simulink model "BEV_Laengsdynamikmodell_v2"  (R2023b)
settings: configuration reference "SharedConfig" (kept outside this file)
undefined symbols (not defined in the file): acc_cycle_flag, Analyse, battery, battery_builder_rtmsupport, config_battery, config_gearbox, config_Inverter, config_motor, config_vehicle, GB, gcbh, gearbox_map, k_FW, ModuleAssembly1, ModuleType1, motormap, motormap2
libraries: powerlib x37, nesl_utility x18, GD_Batterymodel_NSGAII_1_lib x12, BatteryProtection x9, fl_lib x7, dspstat3 x4, simulink x3, eePmsmCurrentReferenceGen x2, spsControlledCurrentSourceLib x2, spsVoltageMeasurementLib x2, batt_lib x1, BatteryBalancing x1
(part 2 of 6)

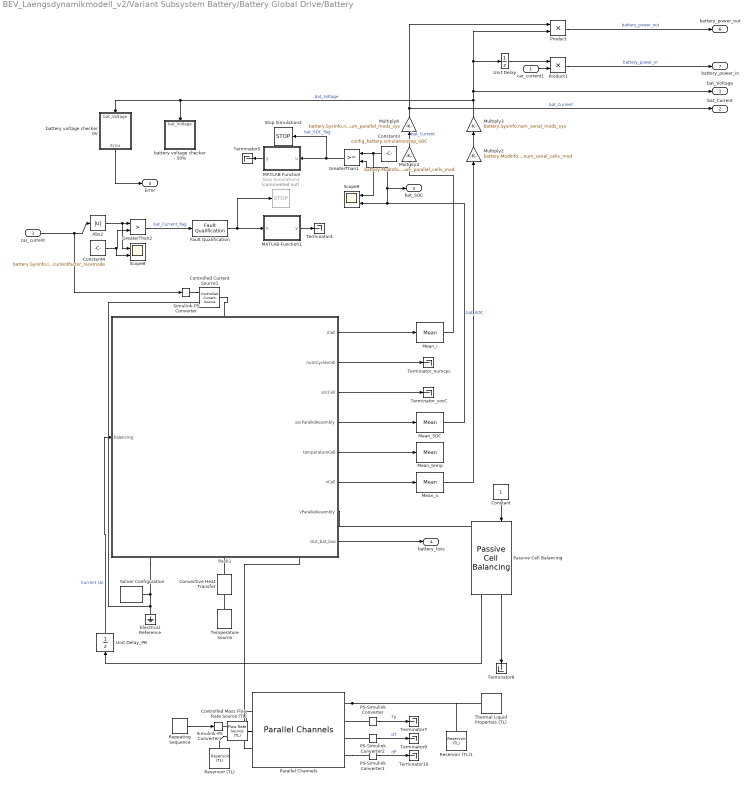
== system BEV_Laengsdynamikmodell_v2/Variant Subsystem Battery/Battery Global Drive/Battery ==
  car_current : Inport
  Abs2 : Abs  SaturateOnIntegerOverflow=off
  Constant : Constant
  Constant3 : Constant  Value=config_battery.simulationstop_SOC
  Constant4 : Constant  Value=battery.SysInfo.I_max_sys * config_battery.overcurrentfactor_racemode
  Controlled Current Source1 : fl_lib/Electrical/Electrical Sources/Controlled Current Source
  Controlled Mass Flow Rate Source (TL) : fl_lib/Thermal Liquid/Sources/Flow Rate Source (TL)  source_type=foundation.enum.constant_controlled.controlled  flow_type=foundation.enum.mass_volumetric_flow.mass  mass_flow=0 kg/s  volumetric_flow=0 m^3/s  power_spec=foundation.enum.power_spec.isentropic  area=0.01 m^2
  Convective Heat Transfer : fl_lib/Thermal/Thermal Elements/Convective Heat Transfer  thermal_type=foundation.enum.constant_variable.constant  area=battery.SysInfo.dim_surface m^2  heat_tr_coeff=20 W/(K*m^2)  min_heat_tr_coeff=1e-3 W/(K*m^2)  T_specify=off  T_priority=None  T=0 K  T_nominal_specify=off  T_nominal_unit=K  T_nominal_value=1  Q_specify=off  Q_priority=None  Q=0 W  Q_nominal_specify=off  Q_nominal_unit=W  Q_nominal_value=1
  Electrical Reference : fl_lib/Electrical/Electrical Elements/Electrical Reference
  Fault Qualification : BatteryProtection/Fault Qualification  QualTime=3  DisqualTime=6  Ts=-1
  GreaterThan1 : RelationalOperator  OutDataTypeStr=boolean  RndMeth=Simplest  InputSameDT=off
  GreaterThan2 : RelationalOperator  Operator=>  OutDataTypeStr=boolean  RndMeth=Simplest  InputSameDT=off
  MATLAB Function : MATLAB Function  TreatAsAtomicUnit=on
  MATLAB Function1 : MATLAB Function  TreatAsAtomicUnit=on
  Mean_SOC : dspstat3/Mean  run=off  InputProcessing=Columns as channels (frame based)  reset_popup=None  directionMode=Entire input  dimension=1  roiEnable=off  roiType=Rectangles  roiPortion=Entire ROI  roiOutput=Individual statistics for each ROI  roiFlag=off  roundingMode=Nearest  overflowMode=off  outputDataTypeStr=Inherit: Same as accumulator  outputMin=[]  outputMax=[]  outputLastDataTypeStr=Inherit: Same as accumulator
  Mean_i : dspstat3/Mean  run=off  InputProcessing=Columns as channels (frame based)  reset_popup=None  directionMode=Entire input  dimension=1  roiEnable=off  roiType=Rectangles  roiPortion=Entire ROI  roiOutput=Individual statistics for each ROI  roiFlag=off  roundingMode=Nearest  overflowMode=off  outputDataTypeStr=Inherit: Same as accumulator  outputMin=[]  outputMax=[]  outputLastDataTypeStr=Inherit: Same as accumulator
  Mean_temp : dspstat3/Mean  run=off  InputProcessing=Columns as channels (frame based)  reset_popup=None  directionMode=Entire input  dimension=1  roiEnable=off  roiType=Rectangles  roiPortion=Entire ROI  roiOutput=Individual statistics for each ROI  roiFlag=off  roundingMode=Nearest  overflowMode=off  outputDataTypeStr=Inherit: Same as accumulator  outputMin=[]  outputMax=[]  outputLastDataTypeStr=Inherit: Same as accumulator
  Mean_v : dspstat3/Mean  run=off  InputProcessing=Columns as channels (frame based)  reset_popup=None  directionMode=Entire input  dimension=1  roiEnable=off  roiType=Rectangles  roiPortion=Entire ROI  roiOutput=Individual statistics for each ROI  roiFlag=off  roundingMode=Nearest  overflowMode=off  outputDataTypeStr=Inherit: Same as accumulator  outputMin=[]  outputMax=[]  outputLastDataTypeStr=Inherit: Same as accumulator
  Multiply2 : Gain  Gain=battery.ModInfo.num_serial_cells_mod
  Multiply3 : Gain  Gain=battery.SysInfo.num_serial_mods_sys
  Multiply4 : Gain  Gain=battery.ModInfo.num_parallel_cells_mod
  Multiply6 : Gain  Gain=battery.SysInfo.num_parallel_mods_sys
  PS-Simulink Converter : nesl_utility/PS-Simulink Converter  PhysicalDomain=network_engine_domain  SubClassName=ps_output  LeftPortType=input  RightPortType=output  PseudoPeriodic=off  Frequencies=[]  VectorFormat=inherit  Unit=inherit  AffineConversion=off
  PS-Simulink Converter1 : nesl_utility/PS-Simulink Converter  PhysicalDomain=network_engine_domain  SubClassName=ps_output  LeftPortType=input  RightPortType=output  PseudoPeriodic=off  Frequencies=[]  VectorFormat=inherit  Unit=inherit  AffineConversion=off
  PS-Simulink Converter2 : nesl_utility/PS-Simulink Converter  PhysicalDomain=network_engine_domain  SubClassName=ps_output  LeftPortType=input  RightPortType=output  PseudoPeriodic=off  Frequencies=[]  VectorFormat=inherit  Unit=inherit  AffineConversion=off
  Pack1 : Subsystem  LoadFcn=battery_builder_rtmsupport('loadfcn',gcbh);
      settings: CopyFcn=battery_builder_rtmsupport('copyfcn',gcbh);  PreCopyFcn=battery_builder_rtmsupport('precopyfcn',gcbh);  PreDeleteFcn=battery_builder_rtmsupport('predeletefcn',gcbh);  PortSchema="{\"entries\":[{\"content\":{\"sides\":[{\"content\":{\"connectorIds\":[\"LConn1\"]},\"type\":\"ConnectorPlacement.EquallySpacedRectSide\",\"uuid\":\"40a787f1-8ebe-41ff-9d70-768a8ef233ef\"},{\"content\":{\"connectorIds\":[\"RConn1\",\"RConn2\",\"RConn3\"],\"side\":\"RIGHT\"},\"type\":\"ConnectorPlacement.EquallySpacedRectSide\",\"uuid\":\"73afe2bc-4ac0-4ad9-926b-4091302672c8\"},{\"content\":{\"connectorIds\":[\"In1\"],\"side\":\"TOP\"},\"type\":\"ConnectorPlacement.EquallySpacedRectSide\",\"uuid\":\"f1f72aa1-a386-4211-9fd1-7dfd903700b9\"},{\"content\":{\"connectorIds\":[\"Out1\",\"Out2\",\"Out3\",\"Out4\",\"Out5\",\"Out6\",\"Out7\",\"Out8\"],\"side\":\"BOTTOM\"},\"type\":\"ConnectorPlacement.EquallySpacedRectSide\",\"uuid\":\"a6cbfe1d-3e62-42c0-b41b-240b72843341\"}]},\"type\":\"ConnectorPlacement.EquallySpacedConnector\",\"uuid\":\"98f8c68d-7fa8-455c-b597-e5213026d8a2\"}],\"packageUris\":[\"http://schema.mathworks.com/mf0/Connector/R2020b\"],\"version\":\"1.0\"}"
      mask Display: image('$imagefile')
  Parallel Channels : batt_lib/Thermal/Parallel Channels  plateConnectivity=simscape.battery.enum.thermal.coolingPlateConnectivity.singleSided  numBattThermalNodes1=1  dimensionThermalNodes1=ones(1, 2)  locationThermalNodes1=ones(1, 2)  numBattThermalNodes2=1  dimensionThermalNodes2=ones(1, 2)  locationThermalNodes2=ones(1, 2)  plateDimX=2  plateDimY=5  plateTh=2e-3 m  plateThCond=20 W/(K*m)  plateDen=2500 kg/m^3  plateCp=447 J/(K*kg)  plateTemp_ini=config_vehicle.ambient_temp K  Re_lam=2000  Re_tur=4000  Nu_lam=3.66  length_add=1e-3 m  shape_factor=64  nChannels=4  selectChannelOrientation=simscape.battery.enum.thermal.coolingChannelsDirection.alongX  channelDia=0.005 m  distributorDia=0.005 m  roughnessPipe=1.5e-05 m
      settings: InternalSimscapePortConfiguration="{\"Bottom\":[],\"Left\":[{\"id\":\"fluid_in\",\"label\":\"fluid_in\",\"type\":\"foundation.thermal_liquid.thermal_liquid\"}],\"Right\":[{\"id\":\"fluid_out\",\"label\":\"fluid_out\",\"type\":\"foundation.thermal_liquid.thermal_liquid\"},{\"id\":\"plotPlateT\",\"label\":\"Tp\",\"type\":\"output\"},{\"id\":\"tempSensor\",\"label\":\"dT\",\"type\":\"output\"},{\"id\":\"presSensor\",\"label\":\"dP\",\"type\":\"output\"}],\"Top\":[{\"id\":\"Side1\",\"label\":\"Surf1\",\"type\":\"foundation.thermal.thermal\"}]}"
  Passive Cell Balancing : BatteryBalancing/Passive Cell Balancing  Threshold=0.2  HysteresisBand=0  Td_on=1  Td_off=1  Ts=-1  dataType=double
  Product : Product
  Product1 : Product
  Repeating Sequence : simulink/Sources/Repeating Sequence  rep_seq_t=[0 2001]  rep_seq_y=[0.1 0.1]
  Reservoir (TL) : fl_lib/Thermal Liquid/Elements/Reservoir (TL)  pressure_spec=foundation.enum.pressure_spec.atmospheric  reservoir_pressure=0.101325 MPa  reservoir_temperature=config_vehicle.ambient_temp K  area=0.01 m^2
  Reservoir (TL)1 : fl_lib/Thermal Liquid/Elements/Reservoir (TL)  pressure_spec=foundation.enum.pressure_spec.atmospheric  reservoir_pressure=0.101325 MPa  reservoir_temperature=config_vehicle.ambient_temp K  area=0.01 m^2
  Scope8 : Scope  NumInputPorts=2
  Scope9 : Scope  NumInputPorts=2
  Simulink-PS Converter : nesl_utility/Simulink-PS Converter  PhysicalDomain=network_engine_domain  SubClassName=ps_input  LeftPortType=input  RightPortType=output  PseudoPeriodic=off  Frequencies=[]  NoiseDistribution=none  NoiseParameters=[]  Unit=1  AffineConversion=off  FilteringAndDerivatives=provide  SimscapeFilterOrder=1  InputFilterTimeConstant=0.001  UdotUserProvided=0
  Simulink-PS Converter1 : nesl_utility/Simulink-PS Converter  PhysicalDomain=network_engine_domain  SubClassName=ps_input  LeftPortType=input  RightPortType=output  PseudoPeriodic=off  Frequencies=[]  NoiseDistribution=none  NoiseParameters=[]  Unit=1  AffineConversion=off  FilteringAndDerivatives=provide  SimscapeFilterOrder=1  InputFilterTimeConstant=0.001  UdotUserProvided=0
  Solver Configuration : nesl_utility/Solver Configuration  PhysicalDomain=network_engine_domain  SubClassName=solver  LeftPortType=input  RightPortType=generic  Tones=[]  Harmonics=[]  SimulateNoise=off  Profile=off  UseLocalSampling=off  EnableSwitchedLinearOptims=on  FrequencyDomain=off  UseCCode=off  RelTol=0.001  AbsTol=0.001  MinStep=1e-09  ToWorkspace=off  RevertToSquareIcSolve=off  NumHomotopyIterations=100  PhasorMode=off  PhasorModeNumHarmonics=1  ConsistencySolver=NEWTON_XTOL_AFTER_FTOL  IndexReductionMethod=DerivativeReplacement  DoDC=off  ResidualTolerance=1e-09  ConsistencyTolSource=GLOBAL  ConsistencyAbsTol=0.001  ConsistencyRelTol=0.001  ConsistencyTolFactor=0.001  UseLocalSolver=on  LocalSolverChoice=NE_BACKWARD_EULER_ADVANCER  ResolveIndetEquations=on  FunctionEvalNumThread=1  LocalSolverSampleTime=1  DoFixedCost=on  MaxNonlinIter=3  MaxModeIter=2  ComputeImpulses=off  ImpulseIterations=2  LinearAlgebra=auto  LinearAlgebraNumThread=0  EquationFormulation=NE_TIME_EF  DelaysMemoryBudget=51200  AutomaticFiltering=on  FilteringTimeConstant=0.001  PartitionStorageMethod=AS_NEEDED  PartitionMemoryBudget=1024  PartitionMethod=ROBUST  MultibodyUseLocalSolver=off  MultibodyLocalSolverChoice=ODE1  MultibodyLocalSolverSampleTime=0.001
  Stop Simulation2 : Stop
  Stop Simulation3 : Stop  Commented=on
  Temperature Source : fl_lib/Thermal/Thermal Sources/Temperature Source  temperature=config_vehicle.ambient_temp K
  Terminator{4..5,7..10} (6 alike) : Terminator
  Terminator_numcyc : Terminator
  Terminator_socC : Terminator
  Thermal Liquid Properties (TL) : SimscapeFluids_lib/Thermal Liquid/Utilities/Thermal Liquid Properties (TL)  fluid_list=fluids.thermal_liquid.utilities.enum.thermal_liquid_fluid_list.water  concentration_param_EG=fluids.thermal_liquid.utilities.enum.thermal_liquid_concentration.volume_fraction  concentration_param_PG=fluids.thermal_liquid.utilities.enum.thermal_liquid_concentration.volume_fraction  c_mass_SW=3.5e-3  c_mass_EG=0.1  c_mass_PG=0.1  c_mass_GL=0.1  c_vol_EG=0.1  c_vol_PG=0.1  beta_const_EG=2.1791 GPa  beta_const_PG=2.1791 GPa  beta_const_GL=2.1791 GPa  p_min_EG=0.01 MPa  p_min_PG=0.01 MPa  p_min_GL=0.01 MPa  p_max_EG=50 MPa  p_max_PG=50 MPa  p_max_GL=50 MPa  p_atm=0.101325 MPa  properties_range_check=simscape.enum.assert.action.error
  Unit Delay : UnitDelay  SampleTime=-1  HasFrameUpgradeWarning=on
  Unit Delay_PB : UnitDelay  SampleTime=-1  HasFrameUpgradeWarning=on
  battery voltage checker - 50% : Subsystem
  battery voltage checker 0V : Subsystem
  car_current1 : InportShadow
  bat_Voltage : Outport
  bat_Current : Outport  Port=2
  bat_SOC : Outport  Port=3
  battery_loss : Outport  Port=4
  Error : Outport  Port=5
  battery_power_out : Outport  Port=6
  battery_power_in : Outport  Port=7
  wires:
  Constant3/1 -> GreaterThan1/1, Scope9/1
  PS-Simulink Converter1/1 -> Terminator10/1  "dP"
  Constant/1 -> Passive Cell Balancing/2
  car_current/1 -> Abs2/1, Simulink-PS Converter/1
  Mean_v/1 -> Multiply2/1
  Multiply3/1 -> bat_Voltage/1, Unit Delay/1, Product/2, battery voltage checker - 50%/1(bat_Voltage), battery voltage checker 0V/1(bat_Voltage)  "bat_Voltage"
  PS-Simulink Converter/1 -> Terminator7/1  "Tp"
  Abs2/1 -> Scope8/1, GreaterThan2/1
  Multiply6/1 -> Product/1, bat_Current/1  "bat_Current"
  Passive Cell Balancing/1 -> Unit Delay_PB/1
  Constant4/1 -> Scope8/2, GreaterThan2/2
  Mean_SOC/1 -> GreaterThan1/2, bat_SOC/1, Scope9/2  "bat_SOC"
  Passive Cell Balancing/2 -> Terminator8/1
  Mean_i/1 -> Multiply4/1
  GreaterThan1/1 -> Stop Simulation2/1, MATLAB Function/1(u)  "bat_SOC_flag"
  GreaterThan2/1 -> Fault Qualification/1  "bat_Current_flag"
  MATLAB Function/1(y) -> Terminator5/1
  MATLAB Function1/1(y) -> Terminator4/1
  Multiply4/1 -> Multiply6/1  "bat_Current"
  battery voltage checker 0V/1(Error) -> Error/1
  Multiply2/1 -> Multiply3/1
  Fault Qualification/1 -> Stop Simulation3/1, MATLAB Function1/1(u)
  Repeating Sequence/1 -> Simulink-PS Converter1/1
  PS-Simulink Converter2/1 -> Terminator9/1  "dT"
  car_current1/1 -> Product1/2
  Unit Delay/1 -> Product1/1
  Product/1 -> battery_power_out/1  "battery_power_out"
  Product1/1 -> battery_power_in/1  "battery_power_in"
  Pack1/1(iCell) -> Mean_i/1
  Pack1/2(numCyclesCell) -> Terminator_numcyc/1
  Pack1/3(socCell) -> Terminator_socC/1
  Pack1/4(socParallelAssembly) -> Mean_SOC/1
  Pack1/5(temperatureCell) -> Mean_temp/1
  Pack1/6(vCell) -> Mean_v/1
  Pack1/7(vParallelAssembly) -> Passive Cell Balancing/1
  Unit Delay_PB/1 -> Pack1/1(balancing)  "Current (A)"
  Pack1/8(Out_bat_loss) -> battery_loss/1
  connections:
  Parallel Channels/RConn1 -- Reservoir (TL)1/LConn1 -- Thermal Liquid Properties (TL)/RConn1
  Temperature Source/LConn1 -- Convective Heat Transfer/RConn1
  Reservoir (TL)/LConn1 -- Controlled Mass Flow Rate Source (TL)/LConn1
  PS-Simulink Converter2/LConn1 -- Parallel Channels/RConn3
  Parallel Channels/RConn4 -- PS-Simulink Converter1/LConn1
  PS-Simulink Converter/LConn1 -- Parallel Channels/RConn2
  Controlled Current Source1/RConn2 -- Electrical Reference/LConn1 -- Solver Configuration/RConn1 -- Pack1/RConn1
  Controlled Mass Flow Rate Source (TL)/RConn1 -- Parallel Channels/LConn1
  Simulink-PS Converter1/RConn1 -- Controlled Mass Flow Rate Source (TL)/LConn2
  Simulink-PS Converter/RConn1 -- Controlled Current Source1/RConn1
  Controlled Current Source1/LConn1 -- Pack1/LConn1
  Pack1/RConn2 -- Convective Heat Transfer/LConn1
  Pack1/RConn3 -- Parallel Channels/LConn2

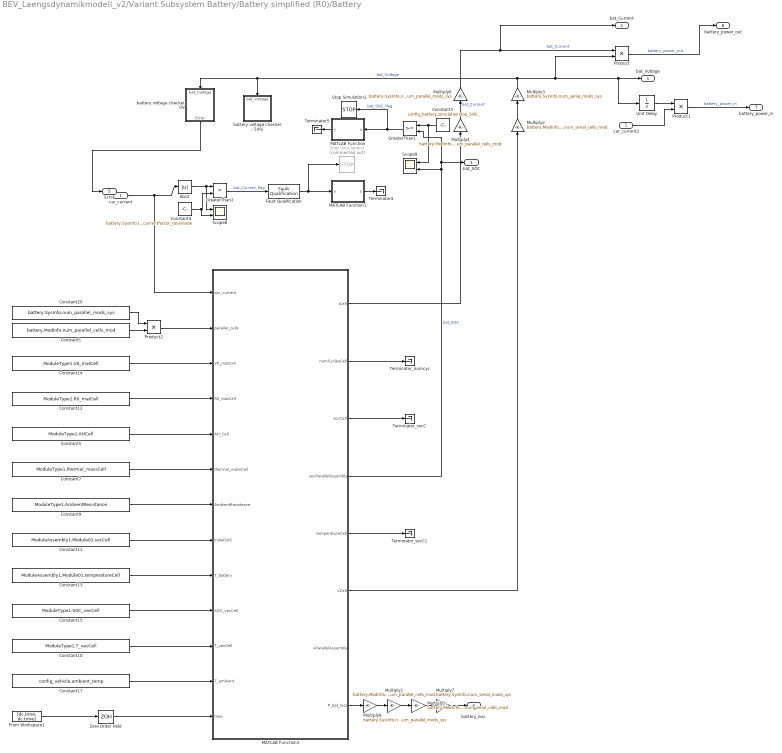
== system BEV_Laengsdynamikmodell_v2/Variant Subsystem Battery/Battery simplified (R0)/Battery ==
  car_current : Inport
  Abs2 : Abs  SaturateOnIntegerOverflow=off
  Constant1 : Constant  Value=battery.ModInfo.num_parallel_cells_mod
  Constant10 : Constant  Value=ModuleType1.T_vecCell
  Constant11 : Constant  Value=ModuleAssembly1.Module01.socCell
  Constant12 : Constant  Value=ModuleType1.R0_matCell
  Constant13 : Constant  Value=ModuleAssembly1.Module01.temperatureCell
  Constant14 : Constant  Value=ModuleType1.V0_matCell
  Constant15 : Constant  Value=ModuleType1.SOC_vecCell
  Constant17 : Constant  Value=config_vehicle.ambient_temp
  Constant20 : Constant  Value=battery.SysInfo.num_parallel_mods_sys
  Constant3 : Constant  Value=config_battery.simulationstop_SOC
  Constant4 : Constant  Value=battery.SysInfo.I_max_sys * config_battery.overcurrentfactor_racemode
  Constant5 : Constant  Value=ModuleType1.AHCell
  Constant7 : Constant  Value=ModuleType1.thermal_massCell
  Constant9 : Constant  Value=ModuleType1.AmbientResistance
  Fault Qualification : BatteryProtection/Fault Qualification  QualTime=3  DisqualTime=6  Ts=-1
  From Workspace1 : FromWorkspace  VariableName=[dc.time, dc.time]
  GreaterThan1 : RelationalOperator  OutDataTypeStr=boolean  RndMeth=Simplest  InputSameDT=off
  GreaterThan2 : RelationalOperator  Operator=>  OutDataTypeStr=boolean  RndMeth=Simplest  InputSameDT=off
  MATLAB Function : MATLAB Function  TreatAsAtomicUnit=on
  MATLAB Function1 : MATLAB Function  TreatAsAtomicUnit=on
  MATLAB Function3 : MATLAB Function  TreatAsAtomicUnit=on
  Multiply1 : Gain  Gain=battery.ModInfo.num_parallel_cells_mod
  Multiply2 : Gain  Gain=battery.ModInfo.num_serial_cells_mod
  Multiply3 : Gain  Gain=battery.SysInfo.num_serial_mods_sys
  Multiply4 : Gain  Gain=battery.ModInfo.num_parallel_cells_mod
  Multiply5 : Gain  Gain=battery.ModInfo.num_serial_cells_mod
  Multiply6 : Gain  Gain=battery.SysInfo.num_parallel_mods_sys
  Multiply7 : Gain  Gain=battery.SysInfo.num_serial_mods_sys
  Multiply8 : Gain  Gain=battery.SysInfo.num_parallel_mods_sys
  Product : Product
  Product1 : Product
  Product2 : Product
  Scope8 : Scope  NumInputPorts=2
  Scope9 : Scope  NumInputPorts=2
  Stop Simulation2 : Stop
  Stop Simulation3 : Stop  Commented=on
  Terminator4 : Terminator
  Terminator5 : Terminator
  Terminator_numcyc : Terminator
  Terminator_socC : Terminator
  Terminator_socC1 : Terminator
  Unit Delay : UnitDelay  SampleTime=-1  HasFrameUpgradeWarning=on
  Zero-Order Hold : ZeroOrderHold  SampleTime=-1
  battery voltage checker - 50% : Subsystem
  battery voltage checker 0V : Subsystem
  car_current2 : InportShadow
  bat_Voltage : Outport
  bat_Current : Outport  Port=2
  bat_SOC : Outport  Port=3
  battery_loss : Outport  Port=4
  Error : Outport  Port=5
  battery_power_out : Outport  Port=6
  battery_power_in : Outport  Port=7
  wires:
  Constant3/1 -> GreaterThan1/1, Scope9/1
  car_current/1 -> MATLAB Function3/1(car_current), Abs2/1
  MATLAB Function3/6(vCell) -> Multiply2/1
  Multiply3/1 -> Product/2, bat_Voltage/1, Unit Delay/1, battery voltage checker - 50%/1(bat_Voltage), battery voltage checker 0V/1(bat_Voltage)  "bat_Voltage"
  Abs2/1 -> Scope8/1, GreaterThan2/1
  Constant4/1 -> Scope8/2, GreaterThan2/2
  MATLAB Function3/4(socParallelAssembly) -> GreaterThan1/2, bat_SOC/1, Scope9/2  "bat_SOC"
  MATLAB Function3/1(iCell) -> Multiply4/1
  GreaterThan1/1 -> Stop Simulation2/1, MATLAB Function/1(u)  "bat_SOC_flag"
  GreaterThan2/1 -> Fault Qualification/1  "bat_Current_flag"
  MATLAB Function/1(y) -> Terminator5/1
  MATLAB Function1/1(y) -> Terminator4/1
  Multiply4/1 -> Multiply6/1  "bat_Current"
  MATLAB Function3/3(socCell) -> Terminator_socC/1
  battery voltage checker 0V/1(Error) -> Error/1
  Multiply2/1 -> Multiply3/1
  Fault Qualification/1 -> Stop Simulation3/1, MATLAB Function1/1(u)
  MATLAB Function3/2(numCyclesCell) -> Terminator_numcyc/1
  MATLAB Function3/5(temperatureCell) -> Terminator_socC1/1
  car_current2/1 -> Product1/2
  Unit Delay/1 -> Product1/1
  Multiply6/1 -> bat_Current/1, Product/1  "bat_Current"
  Product1/1 -> battery_power_in/1  "battery_power_in"
  Product/1 -> battery_power_out/1  "battery_power_out"
  Zero-Order Hold/1 -> MATLAB Function3/13(time)
  From Workspace1/1 -> Zero-Order Hold/1
  Constant5/1 -> MATLAB Function3/5(AH_Cell)
  Constant13/1 -> MATLAB Function3/9(T_battery)
  Constant11/1 -> MATLAB Function3/8(InitialSOC)
  Constant14/1 -> MATLAB Function3/3(V0_matCell)
  Constant12/1 -> MATLAB Function3/4(R0_matCell)
  Constant15/1 -> MATLAB Function3/10(SOC_vecCell)
  Constant7/1 -> MATLAB Function3/6(thermal_massCell)
  Constant10/1 -> MATLAB Function3/11(T_vecCell)
  Constant9/1 -> MATLAB Function3/7(AmbientResistance)
  Constant17/1 -> MATLAB Function3/12(T_ambient)
  Multiply7/1 -> battery_loss/1
  MATLAB Function3/8(P_bat_loss) -> Multiply8/1
  Multiply5/1 -> Multiply7/1
  Multiply1/1 -> Multiply5/1
  Constant1/1 -> Product2/2
  Constant20/1 -> Product2/1
  Product2/1 -> MATLAB Function3/2(parallel_cells)
  Multiply8/1 -> Multiply1/1

== system BEV_Laengsdynamikmodell_v2/Variant Subsystem Gearbox/Gearbox Analytic/Oil Temp ==
  P_V : Inport
  IC : InitialCondition  Value=25
  MATLAB Function : MATLAB Function  TreatAsAtomicUnit=on
  Memory1 : Memory  InitialCondition=config_vehicle.ambient_temp - 273
  Memory2 : Memory  InitialCondition=config_vehicle.ambient_temp - 273
  Scope : Scope
  temp : Outport
  wires:
  MATLAB Function/1(T) -> IC/1  "GB_temp"
  Memory1/1 -> MATLAB Function/1(t)
  P_V/1 -> Memory2/1
  IC/1 -> Scope/1, Memory1/1, temp/1
  Memory2/1 -> MATLAB Function/2(P_V)

== system BEV_Laengsdynamikmodell_v2/Variant Subsystem Gearbox/Gearbox Analytic/Oil Temp Gao ==
  note: entspricht 2pi/60 * 1e-3
  T_wheel : Inport
  rpm_wheel : Inport  Port=2
  MATLAB Function : MATLAB Function  TreatAsAtomicUnit=on
  Memory1 : Memory  InitialCondition=config_vehicle.ambient_temp - 273
  Multiply5 : Gain  Gain=1/9550
  Product2 : Product
  Scope : Scope
  temp : Outport
  wires:
  Product2/1 -> Multiply5/1
  rpm_wheel/1 -> MATLAB Function/3(rpm), Product2/2
  T_wheel/1 -> Product2/1
  MATLAB Function/1(T) -> Scope/1, Memory1/1, temp/1
  Memory1/1 -> MATLAB Function/1(t)
  Multiply5/1 -> MATLAB Function/2(P)

== system BEV_Laengsdynamikmodell_v2/Variant Subsystem Gearbox/Gearbox Analytic/Variant Subsystem Analytic GB ==
  note: 1) Add Subsystem or Model blocks as valid variant choices.
      | 2) You cannot connect blocks at this level. At simulation, connectivity is automatically
      | determined, based on the active variant and port name matching.
  wheel_torque : Inport
  wheel_rpm : Inport  Port=2
  Temp : Inport  Port=3
  Einstufig_Achsparallel : Subsystem  VariantControl=GB_Stufen == 1
  Zweistufig_Achsparallel : Subsystem  VariantControl="GB_Stufen == 2 && GB_Topology == \"achsparallel\""
  Zweistufig_Koaxial : Subsystem  VariantControl="GB_Stufen == 2 && GB_Topology == \"koaxial\""
  P_V : Outport

== system BEV_Laengsdynamikmodell_v2/Variant Subsystem Gearbox/Gearbox Lookup-Table/Oil Temp ==
  P_V : Inport
  IC : InitialCondition  Value=25
  MATLAB Function : MATLAB Function  TreatAsAtomicUnit=on
  Memory1 : Memory  InitialCondition=config_vehicle.ambient_temp - 273
  Memory2 : Memory  InitialCondition=config_vehicle.ambient_temp - 273
  Scope : Scope
  temp : Outport
  wires:
  MATLAB Function/1(T) -> IC/1  "GB_temp"
  Memory1/1 -> MATLAB Function/1(t)
  P_V/1 -> Memory2/1
  IC/1 -> Scope/1, Memory1/1, temp/1
  Memory2/1 -> MATLAB Function/2(P_V)

== system BEV_Laengsdynamikmodell_v2/Variant Subsystem Gearbox/Gearbox Lookup-Table/Oil Temp Gao ==
  note: entspricht 2pi/60 * 1e-3
  T_wheel : Inport
  rpm_wheel : Inport  Port=2
  MATLAB Function : MATLAB Function  TreatAsAtomicUnit=on
  Memory1 : Memory  InitialCondition=config_vehicle.ambient_temp - 273
  Multiply5 : Gain  Gain=1/9550
  Product2 : Product
  Scope : Scope
  temp : Outport
  wires:
  Product2/1 -> Multiply5/1
  rpm_wheel/1 -> MATLAB Function/3(rpm), Product2/2
  T_wheel/1 -> Product2/1
  MATLAB Function/1(T) -> Scope/1, Memory1/1, temp/1
  Memory1/1 -> MATLAB Function/1(t)
  Multiply5/1 -> MATLAB Function/2(P)

== system BEV_Laengsdynamikmodell_v2/Variant Subsystem Gearbox/Gearbox Lookup-Table/Variant Subsystem ==
  note: 1) Add Subsystem or Model blocks as valid variant choices.
      | 2) You cannot connect blocks at this level. At simulation, connectivity is automatically
      | determined, based on the active variant and port name matching.
  wheel_torque : Inport
  wheel_rpm : Inport  Port=2
  Temp : Inport  Port=3
  ETA_map : Subsystem  VariantControl="gearbox_map.map_type == \"Eta\""
  LOSS_map : Subsystem  VariantControl="gearbox_map.map_type == \"Loss\""
  loss_lockup : Outport
  gearbox_efficiency : Outport  Port=2
  gearbox_rpm : Outport  Port=3
  gearbox_torque : Outport  Port=4

== system BEV_Laengsdynamikmodell_v2/Variant Subsystem Inverter/Inverter Analytic/Variant Subsystem ==
  note: 1) Add Subsystem or Model blocks as valid variant choices.
      | 2) You cannot connect blocks at this level. At simulation, connectivity is automatically
      | determined, based on the active variant and port name matching.
  udc : Inport
  rpm : Inport  Port=2
  torque : Inport  Port=3
  terminal_power : Inport  Port=4
  IM_Inverter_IGBT_Analytic : Subsystem  VariantControl=Mode_IM_IGBT
  IM_Inverter_SiC-MOSFET_Analytic : Subsystem  VariantControl=Mode_IM_MOSFET
  PMSM_Inverter_IBGT_Analytic : Subsystem  VariantControl=Mode_PSM_IGBT
  PMSM_Inverter_SiC-MOSFET_Analytic : Subsystem  VariantControl=Mode_PSM_MOSFET
  Conduction_and_Switching_loss : Outport
  idc : Outport  Port=2
  P_inv_total : Outport  Port=3
  P_mot_elec : Outport  Port=4

== system BEV_Laengsdynamikmodell_v2/Variant Subsystem Motor/Motor Analytic/Friction & Windage ==
  note: Gleichung für mechanische Verlustleistung:
      | P_FW = k_FW * n^2.5
  gearbox_rpm : Inport
  Constant : Constant  Value=2.5
  Constant1 : Constant  Value=0
  Constant5 : Constant  Value=k_FW
  Gain : Gain  Gain=2*pi/60
  In2 : InportShadow
  Power : Math  Operator=pow
  Product : Product
  Product2 : Product  Inputs=*/
  Switch : Switch  Criteria=u2 > Threshold  SaturateOnIntegerOverflow=off  InputSameDT=off
  friction torque : Outport
  wires:
  gearbox_rpm/1 -> Power/1  "n_gearbox"
  Constant/1 -> Power/2  "exponent"
  Power/1 -> Product/1
  Constant5/1 -> Product/2
  Product/1 -> Product2/1  "mech powerloss"
  Product2/1 -> Switch/1  "torque"
  In2/1 -> Gain/1  "n_gearbox"
  Gain/1 -> Product2/2, Switch/2
  Switch/1 -> friction torque/1
  Constant1/1 -> Switch/3

== system BEV_Laengsdynamikmodell_v2/Variant Subsystem Motor/Motor Const/Friction & Windage ==
  note: Gleichung für mechanische Verlustleistung:
      | P_FW = k_FW * n^2.5
  gearbox_rpm : Inport
  Constant : Constant  Value=2.5
  Constant1 : Constant  Value=0
  Constant5 : Constant  Value=k_FW
  Gain : Gain  Gain=2*pi/60
  In2 : InportShadow
  Power : Math  Operator=pow
  Product : Product
  Product2 : Product  Inputs=*/
  Switch : Switch  Criteria=u2 > Threshold  SaturateOnIntegerOverflow=off  InputSameDT=off
  friction torque : Outport
  wires:
  gearbox_rpm/1 -> Power/1  "n_gearbox"
  Constant/1 -> Power/2  "exponent"
  Power/1 -> Product/1
  Constant5/1 -> Product/2
  Product/1 -> Product2/1  "mech powerloss"
  Product2/1 -> Switch/1  "torque"
  In2/1 -> Gain/1  "n_gearbox"
  Gain/1 -> Product2/2, Switch/2
  Switch/1 -> friction torque/1
  Constant1/1 -> Switch/3

== system BEV_Laengsdynamikmodell_v2/Variant Subsystem Motor/Motor Lookup-Table/Friction & Windage ==
  note: Gleichung für mechanische Verlustleistung:
      | P_FW = k_FW * n^2.5
  gearbox_rpm : Inport
  Constant : Constant  Value=2.5
  Constant1 : Constant  Value=0
  Constant5 : Constant  Value=k_FW
  Gain : Gain  Gain=2*pi/60
  In2 : InportShadow
  Power : Math  Operator=pow
  Product : Product
  Product2 : Product  Inputs=*/
  Switch : Switch  Criteria=u2 > Threshold  SaturateOnIntegerOverflow=off  InputSameDT=off
  friction torque : Outport
  wires:
  gearbox_rpm/1 -> Power/1  "n_gearbox"
  Constant/1 -> Power/2  "exponent"
  Power/1 -> Product/1
  Constant5/1 -> Product/2
  Product/1 -> Product2/1  "mech powerloss"
  Product2/1 -> Switch/1  "torque"
  In2/1 -> Gain/1  "n_gearbox"
  Gain/1 -> Product2/2, Switch/2
  Switch/1 -> friction torque/1
  Constant1/1 -> Switch/3

== system BEV_Laengsdynamikmodell_v2/Variant Subsystem Motor/Motor Lookup-TableOneMotor/Friction & Windage ==
  note: Gleichung für mechanische Verlustleistung:
      | P_FW = k_FW * n^2.5
  gearbox_rpm : Inport
  Constant : Constant  Value=2.5
  Constant1 : Constant  Value=0
  Constant5 : Constant  Value=k_FW
  Gain : Gain  Gain=2*pi/60
  In2 : InportShadow
  Power : Math  Operator=pow
  Product : Product
  Product2 : Product  Inputs=*/
  Switch : Switch  Criteria=u2 > Threshold  SaturateOnIntegerOverflow=off  InputSameDT=off
  friction torque : Outport
  wires:
  gearbox_rpm/1 -> Power/1  "n_gearbox"
  Constant/1 -> Power/2  "exponent"
  Power/1 -> Product/1
  Constant5/1 -> Product/2
  Product/1 -> Product2/1  "mech powerloss"
  Product2/1 -> Switch/1  "torque"
  In2/1 -> Gain/1  "n_gearbox"
  Gain/1 -> Product2/2, Switch/2
  Switch/1 -> friction torque/1
  Constant1/1 -> Switch/3

== system BEV_Laengsdynamikmodell_v2/Variant Subsystem Battery/Battery Analytic (RC3)/Battery/battery voltage checker - 50% ==
  bat_Voltage : Inport
  Constant : Constant  Value=acc_cycle_flag
  Constant5 : Constant  Value=0.5 * battery.SysInfo.U_max_sys
  Data Type Conversion : DataTypeConversion  OutDataTypeStr=double  SaturateOnIntegerOverflow=off  RndMeth=Floor
  Fault Qualification : BatteryProtection/Fault Qualification  QualTime=2  DisqualTime=4  Ts=-1
  GreaterThan3 : RelationalOperator  Operator=>  OutDataTypeStr=boolean  RndMeth=Simplest  InputSameDT=off
  MATLAB Function2 : MATLAB Function  TreatAsAtomicUnit=on
  Stop Simulation : Stop
  Unit Delay : UnitDelay  SampleTime=-1  HasFrameUpgradeWarning=on
  wires:
  Constant/1 -> MATLAB Function2/3(z)
  Fault Qualification/1 -> MATLAB Function2/1(u)
  MATLAB Function2/2(st) -> Stop Simulation/1
  Data Type Conversion/1 -> MATLAB Function2/2(d)
  Unit Delay/1 -> Data Type Conversion/1
  MATLAB Function2/1(y) -> Unit Delay/1
  bat_Voltage/1 -> GreaterThan3/2
  GreaterThan3/1 -> Fault Qualification/1
  Constant5/1 -> GreaterThan3/1

== system BEV_Laengsdynamikmodell_v2/Variant Subsystem Battery/Battery Analytic (RC3)/Battery/battery voltage checker 0V ==
  bat_Voltage : Inport
  Constant7 : Constant  Value=0
  Fault Qualification1 : BatteryProtection/Fault Qualification  QualTime=1  DisqualTime=3  Ts=-1
  GreaterThan4 : RelationalOperator  Operator=>  OutDataTypeStr=boolean  RndMeth=Simplest  InputSameDT=off
  Error : Outport
  wires:
  Fault Qualification1/1 -> Error/1
  bat_Voltage/1 -> GreaterThan4/2
  GreaterThan4/1 -> Fault Qualification1/1
  Constant7/1 -> GreaterThan4/1

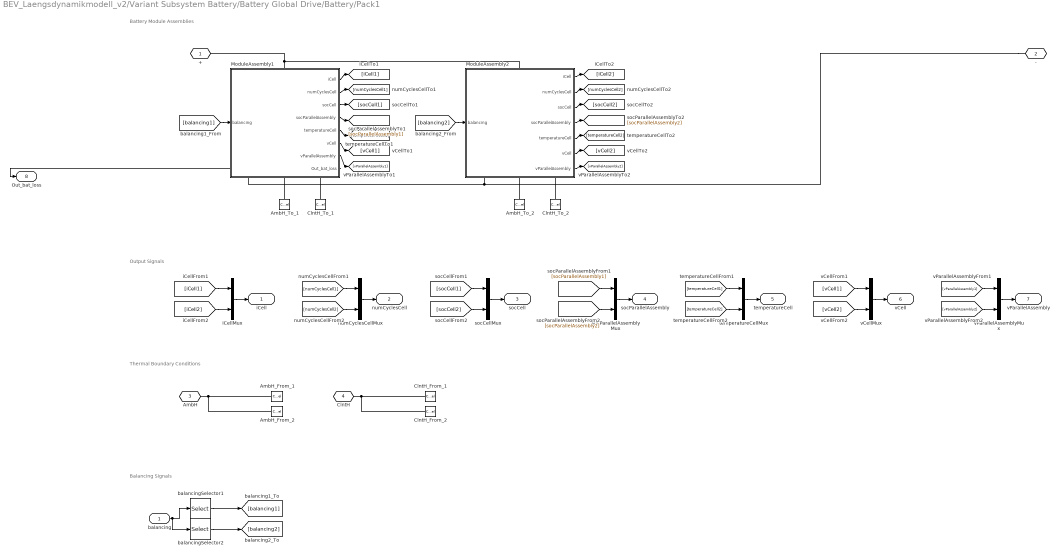
== system BEV_Laengsdynamikmodell_v2/Variant Subsystem Battery/Battery Global Drive/Battery/Pack1 ==
  note: Balancing Signals
  note: Thermal Boundary Conditions
  note: Output Signals
  note: Battery Module Assemblies
  balancing : Inport  PortDimensions=216
  AmbH_From_1 : ConnectionLabel  Label=ambH_1
  AmbH_From_2 : ConnectionLabel  Label=ambH_2
  AmbH_To_1 : ConnectionLabel  Label=ambH_1
  AmbH_To_2 : ConnectionLabel  Label=ambH_2
  ClntH_From_1 : ConnectionLabel  Label=clntH_1
  ClntH_From_2 : ConnectionLabel  Label=clntH_2
  ClntH_To_1 : ConnectionLabel  Label=clntH_1
  ClntH_To_2 : ConnectionLabel  Label=clntH_2
  ModuleAssembly1 : Subsystem  LoadFcn=battery_builder_rtmsupport('loadfcn',gcbh);
      settings: CopyFcn=battery_builder_rtmsupport('copyfcn',gcbh);  PreCopyFcn=battery_builder_rtmsupport('precopyfcn',gcbh);  PreDeleteFcn=battery_builder_rtmsupport('predeletefcn',gcbh);  PortSchema="{\"entries\":[{\"content\":{\"sides\":[{\"content\":{\"connectorIds\":[\"LConn1\"]},\"type\":\"ConnectorPlacement.EquallySpacedRectSide\",\"uuid\":\"40a787f1-8ebe-41ff-9d70-768a8ef233ef\"},{\"content\":{\"connectorIds\":[\"RConn1\",\"RConn2\",\"RConn3\"],\"side\":\"RIGHT\"},\"type\":\"ConnectorPlacement.EquallySpacedRectSide\",\"uuid\":\"73afe2bc-4ac0-4ad9-926b-4091302672c8\"},{\"content\":{\"connectorIds\":[\"In1\"],\"side\":\"TOP\"},\"type\":\"ConnectorPlacement.EquallySpacedRectSide\",\"uuid\":\"f1f72aa1-a386-4211-9fd1-7dfd903700b9\"},{\"content\":{\"connectorIds\":[\"Out1\",\"Out2\",\"Out3\",\"Out4\",\"Out5\",\"Out6\",\"Out7\",\"Out8\"],\"side\":\"BOTTOM\"},\"type\":\"ConnectorPlacement.EquallySpacedRectSide\",\"uuid\":\"00ff99ce-51a0-4b29-8d0f-02bd4eb71b30\"}]},\"type\":\"ConnectorPlacement.EquallySpacedConnector\",\"uuid\":\"98f8c68d-7fa8-455c-b597-e5213026d8a2\"}],\"packageUris\":[\"http://schema.mathworks.com/mf0/Connector/R2020b\"],\"version\":\"1.0\"}"
      mask Display: image('$imagefile')
  ModuleAssembly2 : Subsystem  LoadFcn=battery_builder_rtmsupport('loadfcn',gcbh);
      settings: CopyFcn=battery_builder_rtmsupport('copyfcn',gcbh);  PreCopyFcn=battery_builder_rtmsupport('precopyfcn',gcbh);  PreDeleteFcn=battery_builder_rtmsupport('predeletefcn',gcbh);  PortSchema="{\"entries\":[{\"content\":{\"sides\":[{\"content\":{\"connectorIds\":[\"LConn1\"]},\"type\":\"ConnectorPlacement.EquallySpacedRectSide\",\"uuid\":\"40a787f1-8ebe-41ff-9d70-768a8ef233ef\"},{\"content\":{\"connectorIds\":[\"RConn1\",\"RConn2\",\"RConn3\"],\"side\":\"RIGHT\"},\"type\":\"ConnectorPlacement.EquallySpacedRectSide\",\"uuid\":\"73afe2bc-4ac0-4ad9-926b-4091302672c8\"},{\"content\":{\"connectorIds\":[\"In1\"],\"side\":\"TOP\"},\"type\":\"ConnectorPlacement.EquallySpacedRectSide\",\"uuid\":\"f1f72aa1-a386-4211-9fd1-7dfd903700b9\"},{\"content\":{\"connectorIds\":[\"Out1\",\"Out2\",\"Out3\",\"Out4\",\"Out5\",\"Out6\",\"Out7\"],\"side\":\"BOTTOM\"},\"type\":\"ConnectorPlacement.EquallySpacedRectSide\",\"uuid\":\"00ff99ce-51a0-4b29-8d0f-02bd4eb71b30\"}]},\"type\":\"ConnectorPlacement.EquallySpacedConnector\",\"uuid\":\"98f8c68d-7fa8-455c-b597-e5213026d8a2\"}],\"packageUris\":[\"http://schema.mathworks.com/mf0/Connector/R2020b\"],\"version\":\"1.0\"}"
      mask Display: image('$imagefile')
  balancingSelector1 : Selector  InputPortWidth=216  IndexOptions=Index vector (dialog)  Indices="[1    2    3    4    5    6    7    8    9   10   11   12   13   14   15   16   17   18   19   20   21   22   23   24   25   26   27   28   29   30   31   32   33   34   35   36   37   38   39   40   41   42   43   44   45   46   47   48   49   50   51   52   53   54   55   56   57   58   59   60   61   62   63   64   65   66   67   68   69   70   71   72   73   74   75   76   77   78   79   80   81   82   83   84   85   86   87   88   89   90   91   92   93   94   95   96   97   98   99  100  101  102  103  104  105  106  107  108]"  OutputSizes=1
  balancingSelector2 : Selector  InputPortWidth=216  IndexOptions=Index vector (dialog)  Indices="[109  110  111  112  113  114  115  116  117  118  119  120  121  122  123  124  125  126  127  128  129  130  131  132  133  134  135  136  137  138  139  140  141  142  143  144  145  146  147  148  149  150  151  152  153  154  155  156  157  158  159  160  161  162  163  164  165  166  167  168  169  170  171  172  173  174  175  176  177  178  179  180  181  182  183  184  185  186  187  188  189  190  191  192  193  194  195  196  197  198  199  200  201  202  203  204  205  206  207  208  209  210  211  212  213  214  215  216]"  OutputSizes=1
  iCellMux : Mux  Inputs=2
  numCyclesCellMux : Mux  Inputs=2
  socCellMux : Mux  Inputs=2
  socParallelAssemblyMux : Mux  Inputs=2
  temperatureCellMux : Mux  Inputs=2
  vCellMux : Mux  Inputs=2
  vParallelAssemblyMux : Mux  Inputs=2
  + : PMIOPort  Side=Left
  - : PMIOPort  Port=2  Side=Right
  AmbH : PMIOPort  Port=3  Side=Right  ConnectionType=Connection: foundation.thermal.thermal
  ClntH : PMIOPort  Port=4  Side=Right  ConnectionType=Connection: foundation.thermal.thermal
  iCell : Outport
  numCyclesCell : Outport  Port=2
  socCell : Outport  Port=3
  socParallelAssembly : Outport  Port=4
  temperatureCell : Outport  Port=5
  vCell : Outport  Port=6
  vParallelAssembly : Outport  Port=7
  Out_bat_loss : Outport  Port=8
  wires:
  balancingSelector2/1 -> [balancing2]
  [balancing2] -> ModuleAssembly2/1(balancing)
  balancingSelector1/1 -> [balancing1]
  balancing/1 -> balancingSelector2/1, balancingSelector1/1
  [balancing1] -> ModuleAssembly1/1(balancing)
  [vParallelAssembly2] -> vParallelAssemblyMux/2
  ModuleAssembly2/7(vParallelAssembly) -> [vParallelAssembly2]
  [vCell2] -> vCellMux/2
  ModuleAssembly2/6(vCell) -> [vCell2]
  [temperatureCell2] -> temperatureCellMux/2
  ModuleAssembly2/5(temperatureCell) -> [temperatureCell2]
  [socParallelAssembly2] -> socParallelAssemblyMux/2
  ModuleAssembly2/4(socParallelAssembly) -> [socParallelAssembly2]
  [socCell2] -> socCellMux/2
  ModuleAssembly2/3(socCell) -> [socCell2]
  [numCyclesCell2] -> numCyclesCellMux/2
  ModuleAssembly2/2(numCyclesCell) -> [numCyclesCell2]
  [iCell2] -> iCellMux/2
  ModuleAssembly2/1(iCell) -> [iCell2]
  [vParallelAssembly1] -> vParallelAssemblyMux/1
  vParallelAssemblyMux/1 -> vParallelAssembly/1
  ModuleAssembly1/7(vParallelAssembly) -> [vParallelAssembly1]
  [vCell1] -> vCellMux/1
  vCellMux/1 -> vCell/1
  ModuleAssembly1/6(vCell) -> [vCell1]
  [temperatureCell1] -> temperatureCellMux/1
  temperatureCellMux/1 -> temperatureCell/1
  ModuleAssembly1/5(temperatureCell) -> [temperatureCell1]
  [socParallelAssembly1] -> socParallelAssemblyMux/1
  socParallelAssemblyMux/1 -> socParallelAssembly/1
  ModuleAssembly1/4(socParallelAssembly) -> [socParallelAssembly1]
  [socCell1] -> socCellMux/1
  socCellMux/1 -> socCell/1
  ModuleAssembly1/3(socCell) -> [socCell1]
  [numCyclesCell1] -> numCyclesCellMux/1
  numCyclesCellMux/1 -> numCyclesCell/1
  ModuleAssembly1/2(numCyclesCell) -> [numCyclesCell1]
  [iCell1] -> iCellMux/1
  iCellMux/1 -> iCell/1
  ModuleAssembly1/1(iCell) -> [iCell1]
  ModuleAssembly1/8(Out_bat_loss) -> Out_bat_loss/1
  connections:
  ClntH_To_2/LConn1 -- ModuleAssembly2/RConn3
  ClntH_From_2/LConn1 -- ClntH_From_1/LConn1 -- ClntH/RConn1
  ClntH_To_1/LConn1 -- ModuleAssembly1/RConn3
  AmbH_To_2/LConn1 -- ModuleAssembly2/RConn2
  AmbH_From_2/LConn1 -- AmbH_From_1/LConn1 -- AmbH/RConn1
  AmbH_To_1/LConn1 -- ModuleAssembly1/RConn2
  -/RConn1 -- ModuleAssembly2/RConn1 -- ModuleAssembly1/RConn1
  +/RConn1 -- ModuleAssembly2/LConn1 -- ModuleAssembly1/LConn1

== system BEV_Laengsdynamikmodell_v2/Variant Subsystem Battery/Battery Global Drive/Battery/battery voltage checker - 50% ==
  bat_Voltage : Inport
  Constant : Constant  Value=acc_cycle_flag
  Constant5 : Constant  Value=0.5 * battery.SysInfo.U_max_sys
  Data Type Conversion : DataTypeConversion  OutDataTypeStr=double  SaturateOnIntegerOverflow=off  RndMeth=Floor
  Fault Qualification : BatteryProtection/Fault Qualification  QualTime=2  DisqualTime=4  Ts=-1
  GreaterThan3 : RelationalOperator  Operator=>  OutDataTypeStr=boolean  RndMeth=Simplest  InputSameDT=off
  MATLAB Function2 : MATLAB Function  TreatAsAtomicUnit=on
  Stop Simulation : Stop
  Unit Delay : UnitDelay  SampleTime=-1  HasFrameUpgradeWarning=on
  wires:
  Constant5/1 -> GreaterThan3/1
  GreaterThan3/1 -> Fault Qualification/1
  bat_Voltage/1 -> GreaterThan3/2
  MATLAB Function2/1(y) -> Unit Delay/1
  Unit Delay/1 -> Data Type Conversion/1
  Data Type Conversion/1 -> MATLAB Function2/2(d)
  MATLAB Function2/2(st) -> Stop Simulation/1
  Fault Qualification/1 -> MATLAB Function2/1(u)
  Constant/1 -> MATLAB Function2/3(z)

== system BEV_Laengsdynamikmodell_v2/Variant Subsystem Battery/Battery Global Drive/Battery/battery voltage checker 0V ==
  bat_Voltage : Inport
  Constant7 : Constant  Value=0
  Fault Qualification1 : BatteryProtection/Fault Qualification  QualTime=1  DisqualTime=3  Ts=-1
  GreaterThan4 : RelationalOperator  Operator=>  OutDataTypeStr=boolean  RndMeth=Simplest  InputSameDT=off
  Error : Outport
  wires:
  Constant7/1 -> GreaterThan4/1
  GreaterThan4/1 -> Fault Qualification1/1
  bat_Voltage/1 -> GreaterThan4/2
  Fault Qualification1/1 -> Error/1

== system BEV_Laengsdynamikmodell_v2/Variant Subsystem Battery/Battery simplified (R0)/Battery/battery voltage checker - 50% ==
  bat_Voltage : Inport
  Constant : Constant  Value=acc_cycle_flag
  Constant5 : Constant  Value=0.5 * battery.SysInfo.U_max_sys
  Data Type Conversion : DataTypeConversion  OutDataTypeStr=double  SaturateOnIntegerOverflow=off  RndMeth=Floor
  Fault Qualification : BatteryProtection/Fault Qualification  QualTime=2  DisqualTime=4  Ts=-1
  GreaterThan3 : RelationalOperator  Operator=>  OutDataTypeStr=boolean  RndMeth=Simplest  InputSameDT=off
  MATLAB Function2 : MATLAB Function  TreatAsAtomicUnit=on
  Stop Simulation : Stop
  Unit Delay : UnitDelay  SampleTime=-1  HasFrameUpgradeWarning=on
  wires:
  Constant5/1 -> GreaterThan3/1
  GreaterThan3/1 -> Fault Qualification/1
  bat_Voltage/1 -> GreaterThan3/2
  MATLAB Function2/1(y) -> Unit Delay/1
  Unit Delay/1 -> Data Type Conversion/1
  Data Type Conversion/1 -> MATLAB Function2/2(d)
  MATLAB Function2/2(st) -> Stop Simulation/1
  Fault Qualification/1 -> MATLAB Function2/1(u)
  Constant/1 -> MATLAB Function2/3(z)

== system BEV_Laengsdynamikmodell_v2/Variant Subsystem Battery/Battery simplified (R0)/Battery/battery voltage checker 0V ==
  bat_Voltage : Inport
  Constant7 : Constant  Value=0
  Fault Qualification1 : BatteryProtection/Fault Qualification  QualTime=1  DisqualTime=3  Ts=-1
  GreaterThan4 : RelationalOperator  Operator=>  OutDataTypeStr=boolean  RndMeth=Simplest  InputSameDT=off
  Error : Outport
  wires:
  Constant7/1 -> GreaterThan4/1
  GreaterThan4/1 -> Fault Qualification1/1
  bat_Voltage/1 -> GreaterThan4/2
  Fault Qualification1/1 -> Error/1

== system BEV_Laengsdynamikmodell_v2/Variant Subsystem Gearbox/Gearbox Analytic/Variant Subsystem Analytic GB/Einstufig_Achsparallel ==
  wheel_torque : Inport
  wheel_rpm : Inport  Port=2
  Temp : Inport  Port=3
  Add : Sum
  MATLAB Function : MATLAB Function  TreatAsAtomicUnit=on
  Ölpumpe : Subsystem
  P_V : Outport
  wires:
  wheel_rpm/1 -> Ölpumpe/1(nrad), MATLAB Function/2(nrad)
  MATLAB Function/1(P_V) -> Add/1
  wheel_torque/1 -> MATLAB Function/1(Mrad)
  Temp/1 -> MATLAB Function/3(Temp)
  Add/1 -> P_V/1
  Ölpumpe/1(power_oilpump) -> Add/2

== system BEV_Laengsdynamikmodell_v2/Variant Subsystem Gearbox/Gearbox Analytic/Variant Subsystem Analytic GB/Zweistufig_Achsparallel ==
  wheel_torque : Inport
  wheel_rpm : Inport  Port=2
  Temp : Inport  Port=3
  Add : Sum
  MATLAB Function : MATLAB Function  TreatAsAtomicUnit=on
  Ölpumpe : Subsystem
  P_V : Outport
  wires:
  wheel_rpm/1 -> Ölpumpe/1(nrad), MATLAB Function/2(nrad)
  MATLAB Function/1(P_V) -> Add/1
  wheel_torque/1 -> MATLAB Function/1(Mrad)
  Temp/1 -> MATLAB Function/3(Temp)
  Add/1 -> P_V/1
  Ölpumpe/1(power_oilpump) -> Add/2

== system BEV_Laengsdynamikmodell_v2/Variant Subsystem Gearbox/Gearbox Analytic/Variant Subsystem Analytic GB/Zweistufig_Koaxial ==
  wheel_torque : Inport
  wheel_rpm : Inport  Port=2
  Temp : Inport  Port=3
  Add : Sum
  MATLAB Function : MATLAB Function  TreatAsAtomicUnit=on
  Ölpumpe : Subsystem
  P_V : Outport
  wires:
  Temp/1 -> MATLAB Function/3(Temp)
  wheel_torque/1 -> MATLAB Function/1(Mrad)
  MATLAB Function/1(P_V) -> Add/1
  wheel_rpm/1 -> Ölpumpe/1(nrad), MATLAB Function/2(nrad)
  Add/1 -> P_V/1
  Ölpumpe/1(power_oilpump) -> Add/2

== system BEV_Laengsdynamikmodell_v2/Variant Subsystem Gearbox/Gearbox Lookup-Table/Variant Subsystem/ETA_map ==
  note: Sonderfall: Stillstand
  note: Sonderfall: Stillstand
  note: Wirkungsgrad:
      | Antriebsfall
  note: Wirkungsgrad:
      | Rekuperation
  wheel_torque : Inport
  wheel_rpm : Inport  Port=2
  Temp : Inport  Port=3
  Add1 : Sum
  Add2 : Sum
  Constant5 : Constant  Value=100
  Constant6 : Constant
  Constant9 : Constant  Value=100
  Divide : Product  Inputs=/*
  Divide1 : Product  Inputs=/*
  Divide2 : Product  Inputs=*/
  Divide3 : Product  Inputs=*/
  Divide6 : Product  Inputs=*/
  Gain : Gain  Gain=2*pi/60
  Gain1 : Gain  Gain=2*pi/60
  Gearbox Ratio : Gain  Gain=config_gearbox.iges
  Lookup Gearbox : Subsystem  Variant=on
  Oilpump : Subsystem
  Product2 : Product  Inputs=**
  Product3 : Product  Inputs=**
  Saturation : Saturate  UpperLimit=inf  LowerLimit=0
  Subtract1 : Sum  Inputs=+-
  Switch : Switch  SaturateOnIntegerOverflow=off  InputSameDT=off
  Switch2 : Switch  Criteria=u2 > Threshold  SaturateOnIntegerOverflow=off  InputSameDT=off
  Switch3 : Switch  Criteria=u2 ~= 0  SaturateOnIntegerOverflow=off  InputSameDT=off
  Switch4 : Switch  Criteria=u2 ~= 0  SaturateOnIntegerOverflow=off  InputSameDT=off
  Zero : Constant  Value=0  OutDataTypeStr=Inherit: Inherit via back propagation
  Zero1 : Constant  Value=0  OutDataTypeStr=Inherit: Inherit via back propagation
  loss_lockup : Outport
  gearbox_efficiency : Outport  Port=2
  gearbox_rpm : Outport  Port=3
  gearbox_torque : Outport  Port=4
  wires:
  wheel_torque/1 -> Lookup Gearbox/1(Torque), Switch/2, Product2/1  "wheel_torque"
  Divide1/1 -> Switch2/3
  Product2/1 -> Gain/1
  wheel_rpm/1 -> Switch3/2, Gearbox Ratio/1, Product2/2, Oilpump/1(rpm_wheel), Lookup Gearbox/2(RPM)  "wheel_rpm"
  Constant6/1 -> Subtract1/2
  Subtract1/1 -> Product3/1
  Switch/1 -> Subtract1/1  "efficiency_%"
  Product3/1 -> Add1/1  "powerloss_gear"
  Zero1/1 -> Switch3/3
  Switch2/1 -> Saturation/1
  Divide2/1 -> Switch/1
  Zero/1 -> Switch4/3
  Switch4/1 -> gearbox_torque/1
  Switch3/1 -> gearbox_efficiency/1
  Divide6/1 -> Switch4/1
  Gearbox Ratio/1 -> Gain1/1, gearbox_rpm/1  "gearbox_rpm"
  Divide3/1 -> Switch/3
  Add2/1 -> Switch2/2, Divide6/1, Divide1/2, Divide/1  "gearbox_power"
  Gain1/1 -> Switch4/2, Divide6/2
  Temp/1 -> Lookup Gearbox/3(Temp)
  Gain/1 -> Product3/2, Divide1/1, Divide/2, Add2/2  "wheel_power"
  Add1/1 -> Add2/1, loss_lockup/1  "powerloss_gearbox"
  Constant9/1 -> Divide3/2
  Oilpump/1(loss_oilpump) -> Add1/2  "powerloss_oilpump"
  Lookup Gearbox/1(Eta) -> Divide2/2, Divide3/1
  Divide/1 -> Switch2/1
  Constant5/1 -> Divide2/1
  Saturation/1 -> Switch3/1

== system BEV_Laengsdynamikmodell_v2/Variant Subsystem Gearbox/Gearbox Lookup-Table/Variant Subsystem/LOSS_map ==
  note: Sonderfall: Stillstand
  note: Wirkungsgrad: Antriebsfall
  note: Wirkungsgrad: Rekuperation
  note: Sonderfall: Stillstand
  wheel_torque : Inport
  wheel_rpm : Inport  Port=2
  Temp : Inport  Port=3
  Add1 : Sum
  Add2 : Sum
  Divide : Product  Inputs=/*
  Divide1 : Product  Inputs=/*
  Divide6 : Product  Inputs=*/
  Gain : Gain  Gain=2*pi/60
  Gain1 : Gain  Gain=2*pi/60
  Gearbox Ratio : Gain  Gain=config_gearbox.iges
  Lookup Gearbox : Subsystem  Variant=on
  Oilpump : Subsystem
  Product2 : Product  Inputs=**
  Saturation : Saturate  UpperLimit=inf  LowerLimit=0
  Switch2 : Switch  Criteria=u2 > Threshold  SaturateOnIntegerOverflow=off  InputSameDT=off
  Switch3 : Switch  Criteria=u2 ~= 0  SaturateOnIntegerOverflow=off  InputSameDT=off
  Switch4 : Switch  Criteria=u2 ~= 0  SaturateOnIntegerOverflow=off  InputSameDT=off
  Zero : Constant  Value=0  OutDataTypeStr=Inherit: Inherit via back propagation
  Zero1 : Constant  Value=0  OutDataTypeStr=Inherit: Inherit via back propagation
  loss_lockup : Outport
  gearbox_efficiency : Outport  Port=2
  gearbox_rpm : Outport  Port=3
  gearbox_torque : Outport  Port=4
  wires:
  Gain/1 -> Divide1/1, Divide/2, Add2/2  "wheel_power"
  wheel_torque/1 -> Lookup Gearbox/1(Torque), Product2/1  "wheel_torque"
  Lookup Gearbox/1(Loss) -> Add1/1  "powerloss_gear"
  Product2/1 -> Gain/1
  Switch4/1 -> gearbox_torque/1
  Switch3/1 -> gearbox_efficiency/1
  Gearbox Ratio/1 -> gearbox_rpm/1, Gain1/1  "gearbox_rpm"
  Switch2/1 -> Saturation/1
  Divide/1 -> Switch2/1
  Add2/1 -> Divide/1, Switch2/2, Divide1/2, Divide6/1  "gearbox_power"
  Zero/1 -> Switch4/3
  Divide6/1 -> Switch4/1
  Divide1/1 -> Switch2/3
  Oilpump/1(loss_oilpump) -> Add1/2  "powerloss_oilpump"
  Add1/1 -> loss_lockup/1, Add2/1  "powerloss_gearbox"
  Temp/1 -> Lookup Gearbox/3(Temp)
  Gain1/1 -> Switch4/2, Divide6/2
  wheel_rpm/1 -> Switch3/2, Gearbox Ratio/1, Product2/2, Lookup Gearbox/2(RPM), Oilpump/1(rpm_wheel)  "wheel_rpm"
  Zero1/1 -> Switch3/3
  Saturation/1 -> Switch3/1
